simulink library "AEMS_Standard_Library"  (R2016b)
settings: Solver=ode45  StartTime=0.0  StopTime=10.0  RelTol=1e-3
undefined symbols (not defined in the file or in its folder): BkPY, carto, Cbx_extegr, Cbx_lpegrsys, Cbx_portegr, Cnx_bnk_nr_conf, Cnx_cyl_nr_conf, ConfigManagement, configuration_management, Cxx_dcm_io_tmr_end_xxxx, Cxx_dcm_rt_tmr_end, Cxx_DID_xxxx_IO_max, Cxx_DID_xxxx_IO_min, Cxx_egrhsofs, Cxx_vmaniegi, DEM_DEBOUNCE_FREEZE, DEM_DTR_CTL_INVISIBLE, DEM_DTR_CTL_NORMAL, Dem_DtrId2_XXX, Dem_DtrId3_XXX, Dem_DtrId4_XXX, Dem_DtrId5_XXX, Dem_DtrId6_XXX, Dem_DtrId7_XXX, Dem_DtrId8_XXX, Dem_DtrId9_XXX, Dem_DtrId_XXX, Dem_EnableConditionId2_XXX, Dem_EnableConditionId3_XXX, Dem_EnableConditionId4_XXX, Dem_EnableConditionId5_XXX, Dem_EnableConditionId6_XXX, Dem_EnableConditionId7_XXX, Dem_EnableConditionId8_XXX, Dem_EnableConditionId_XXX, Dem_EventId, Dem_EventId2_XXX, Dem_EventId3_XXX, Dem_EventId4_XXX, Dem_EventId5_XXX, Dem_EventId6_XXX, Dem_EventId7_XXX, Dem_EventId8_XXX, Dem_EventId9_XXX, Dem_EventId_Device_Faulttype, Dem_EventId_XXX, DEM_IUMPR_GENERAL_DENOMINATOR, DEM_OPCYC_IGNITION, Dem_RatioId2_XXX, Dem_RatioId3_XXX, Dem_RatioId4_XXX, Dem_RatioId5_XXX, Dem_RatioId6_XXX, Dem_RatioId7_XXX, Dem_RatioId8_XXX, Dem_RatioId_XXX, Dem_StorageConditionId2_XXX, Dem_StorageConditionId3_XXX, Dem_StorageConditionId4_XXX, Dem_StorageConditionId5_XXX ... (+65)
libraries: AEMS_Standard_Library x477, simulink x2
(part 23 of 39)

== system AEMS_Standard_Library/SUB/AEMS_DEM_REP_IUMPR_8D ==
  denlock_status : Inport
  faultdetect_trigger : Inport  Port=2
  AEMS_EDGE_FALLING : AEMS_Standard_Library/EDGE/AEMS_EDGE_FALLING  Tag=[LIB]  init=false
      settings: AttributesFormatString=|
      | %<MaskType>
      | Initial Value : %<init>
  AEMS_EDGE_RISING1 : AEMS_Standard_Library/EDGE/AEMS_EDGE_RISING  Tag=[LIB]  init=false
      settings: AttributesFormatString=|
      | %<MaskType>
      | Initial Value : %<init>
  AEMS_EDGE_RISING2 : AEMS_Standard_Library/EDGE/AEMS_EDGE_RISING  Tag=[LIB]  init=false
      settings: AttributesFormatString=|
      | %<MaskType>
      | Initial Value : %<init>
  Dem_RepIUMPRDenLock_Call1 : Subsystem  TreatAsAtomicUnit=on
  Dem_RepIUMPRDenLock_Call2 : Subsystem  TreatAsAtomicUnit=on
  Dem_RepIUMPRDenLock_Call3 : Subsystem  TreatAsAtomicUnit=on
  Dem_RepIUMPRDenLock_Call4 : Subsystem  TreatAsAtomicUnit=on
  Dem_RepIUMPRDenLock_Call5 : Subsystem  TreatAsAtomicUnit=on
  Dem_RepIUMPRDenLock_Call6 : Subsystem  TreatAsAtomicUnit=on
  Dem_RepIUMPRDenLock_Call7 : Subsystem  TreatAsAtomicUnit=on
  Dem_RepIUMPRDenLock_Call8 : Subsystem  TreatAsAtomicUnit=on
  Dem_RepIUMPRDenRelease_Call1 : Subsystem  TreatAsAtomicUnit=on
  Dem_RepIUMPRDenRelease_Call2 : Subsystem  TreatAsAtomicUnit=on
  Dem_RepIUMPRDenRelease_Call3 : Subsystem  TreatAsAtomicUnit=on
  Dem_RepIUMPRDenRelease_Call4 : Subsystem  TreatAsAtomicUnit=on
  Dem_RepIUMPRDenRelease_Call5 : Subsystem  TreatAsAtomicUnit=on
  Dem_RepIUMPRDenRelease_Call6 : Subsystem  TreatAsAtomicUnit=on
  Dem_RepIUMPRDenRelease_Call7 : Subsystem  TreatAsAtomicUnit=on
  Dem_RepIUMPRDenRelease_Call8 : Subsystem  TreatAsAtomicUnit=on
  Dem_RepIUMPRFaultDetect_Call1 : Subsystem  TreatAsAtomicUnit=on
  Dem_RepIUMPRFaultDetect_Call2 : Subsystem  TreatAsAtomicUnit=on
  Dem_RepIUMPRFaultDetect_Call3 : Subsystem  TreatAsAtomicUnit=on
  Dem_RepIUMPRFaultDetect_Call4 : Subsystem  TreatAsAtomicUnit=on
  Dem_RepIUMPRFaultDetect_Call5 : Subsystem  TreatAsAtomicUnit=on
  Dem_RepIUMPRFaultDetect_Call6 : Subsystem  TreatAsAtomicUnit=on
  Dem_RepIUMPRFaultDetect_Call7 : Subsystem  TreatAsAtomicUnit=on
  Dem_RepIUMPRFaultDetect_Call8 : Subsystem  TreatAsAtomicUnit=on
  Demux : Demux  Outputs=8
  Demux1 : Demux  Outputs=8
  Demux2 : Demux  Outputs=8
  wires:
  AEMS_EDGE_RISING1/1 -> Demux1/1  "denlock_call"
  AEMS_EDGE_RISING2/1 -> Demux/1  "faultdetect_call"
  AEMS_EDGE_FALLING/1 -> Demux2/1  "denrelease_call"
  Demux2/8 -> Dem_RepIUMPRDenRelease_Call8/Enable  "denrelease_call8"
  Demux2/7 -> Dem_RepIUMPRDenRelease_Call7/Enable  "denrelease_call7"
  Demux2/6 -> Dem_RepIUMPRDenRelease_Call6/Enable  "denrelease_call6"
  Demux2/5 -> Dem_RepIUMPRDenRelease_Call5/Enable  "denrelease_call5"
  Demux2/4 -> Dem_RepIUMPRDenRelease_Call4/Enable  "denrelease_call4"
  Demux2/3 -> Dem_RepIUMPRDenRelease_Call3/Enable  "denrelease_call3"
  Demux2/2 -> Dem_RepIUMPRDenRelease_Call2/Enable  "denrelease_call2"
  Demux2/1 -> Dem_RepIUMPRDenRelease_Call1/Enable  "denrelease_call1"
  Demux1/8 -> Dem_RepIUMPRDenLock_Call8/Enable  "denlock_call8"
  Demux1/7 -> Dem_RepIUMPRDenLock_Call7/Enable  "denlock_call7"
  Demux1/6 -> Dem_RepIUMPRDenLock_Call6/Enable  "denlock_call6"
  Demux1/5 -> Dem_RepIUMPRDenLock_Call5/Enable  "denlock_call5"
  Demux1/4 -> Dem_RepIUMPRDenLock_Call4/Enable  "denlock_call4"
  Demux1/3 -> Dem_RepIUMPRDenLock_Call3/Enable  "denlock_call3"
  Demux1/2 -> Dem_RepIUMPRDenLock_Call2/Enable  "denlock_call2"
  Demux1/1 -> Dem_RepIUMPRDenLock_Call1/Enable  "denlock_call1"
  denlock_status/1 -> AEMS_EDGE_RISING1/1, AEMS_EDGE_FALLING/1  "denlock_status"
  Demux/8 -> Dem_RepIUMPRFaultDetect_Call8/Enable  "faultdetect_call8"
  Demux/7 -> Dem_RepIUMPRFaultDetect_Call7/Enable  "faultdetect_call7"
  Demux/6 -> Dem_RepIUMPRFaultDetect_Call6/Enable  "faultdetect_call6"
  Demux/5 -> Dem_RepIUMPRFaultDetect_Call5/Enable  "faultdetect_call5"
  Demux/4 -> Dem_RepIUMPRFaultDetect_Call4/Enable  "faultdetect_call4"
  Demux/3 -> Dem_RepIUMPRFaultDetect_Call3/Enable  "faultdetect_call3"
  Demux/2 -> Dem_RepIUMPRFaultDetect_Call2/Enable  "faultdetect_call2"
  Demux/1 -> Dem_RepIUMPRFaultDetect_Call1/Enable  "faultdetect_call1"
  faultdetect_trigger/1 -> AEMS_EDGE_RISING2/1  "faultdetect_trigger"

== system AEMS_Standard_Library/SUB/AEMS_DEM_REP_IUMPR_DEN_RELEASE_1D ==
  denlock_status : Inport  OutDataTypeStr=boolean  PortDimensions=1
  AEMS_EDGE_RISING1 : AEMS_Standard_Library/EDGE/AEMS_EDGE_RISING  Tag=[LIB]  init=false
      settings: AttributesFormatString=|
      | %<MaskType>
      | Initial Value : %<init>
  Dem_RepIUMPRDenRelease_call : Subsystem  TreatAsAtomicUnit=on
  wires:
  denlock_status/1 -> AEMS_EDGE_RISING1/1  "denlock_status"
  AEMS_EDGE_RISING1/1 -> Dem_RepIUMPRDenRelease_call/Enable  "denrelease_call"

== system AEMS_Standard_Library/SUB/AEMS_DEM_REP_IUMPR_DEN_RELEASE_2D ==
  denlock_status : Inport  OutDataTypeStr=boolean
  AEMS_EDGE_RISING2 : AEMS_Standard_Library/EDGE/AEMS_EDGE_RISING  Tag=[LIB]  init=false
      settings: AttributesFormatString=|
      | %<MaskType>
      | Initial Value : %<init>
  Dem_RepIUMPRDenRelease_call1 : Subsystem  TreatAsAtomicUnit=on
  Dem_RepIUMPRDenRelease_call2 : Subsystem  TreatAsAtomicUnit=on
  Demux1 : Demux  Outputs=2
  wires:
  Demux1/2 -> Dem_RepIUMPRDenRelease_call2/Enable  "denrelease_call2"
  Demux1/1 -> Dem_RepIUMPRDenRelease_call1/Enable  "denrelease_call1"
  AEMS_EDGE_RISING2/1 -> Demux1/1  "denrelease_call"
  denlock_status/1 -> AEMS_EDGE_RISING2/1  "denlock_status"

== system AEMS_Standard_Library/SUB/AEMS_DEM_REP_IUMPR_DEN_RELEASE_8D ==
  denlock_status : Inport  OutDataTypeStr=boolean
  AEMS_EDGE_RISING1 : AEMS_Standard_Library/EDGE/AEMS_EDGE_RISING  Tag=[LIB]  init=false
      settings: AttributesFormatString=|
      | %<MaskType>
      | Initial Value : %<init>
  Dem_RepIUMPRDenRelease_call1 : Subsystem  TreatAsAtomicUnit=on
  Dem_RepIUMPRDenRelease_call2 : Subsystem  TreatAsAtomicUnit=on
  Dem_RepIUMPRDenRelease_call3 : Subsystem  TreatAsAtomicUnit=on
  Dem_RepIUMPRDenRelease_call4 : Subsystem  TreatAsAtomicUnit=on
  Dem_RepIUMPRDenRelease_call5 : Subsystem  TreatAsAtomicUnit=on
  Dem_RepIUMPRDenRelease_call6 : Subsystem  TreatAsAtomicUnit=on
  Dem_RepIUMPRDenRelease_call7 : Subsystem  TreatAsAtomicUnit=on
  Dem_RepIUMPRDenRelease_call8 : Subsystem  TreatAsAtomicUnit=on
  Demux1 : Demux  Outputs=8
  wires:
  AEMS_EDGE_RISING1/1 -> Demux1/1  "denrelease_call"
  Demux1/8 -> Dem_RepIUMPRDenRelease_call8/Enable  "denrelease_call8"
  Demux1/7 -> Dem_RepIUMPRDenRelease_call7/Enable  "denrelease_call7"
  Demux1/6 -> Dem_RepIUMPRDenRelease_call6/Enable  "denrelease_call6"
  Demux1/5 -> Dem_RepIUMPRDenRelease_call5/Enable  "denrelease_call5"
  Demux1/4 -> Dem_RepIUMPRDenRelease_call4/Enable  "denrelease_call4"
  Demux1/3 -> Dem_RepIUMPRDenRelease_call3/Enable  "denrelease_call3"
  Demux1/2 -> Dem_RepIUMPRDenRelease_call2/Enable  "denrelease_call2"
  Demux1/1 -> Dem_RepIUMPRDenRelease_call1/Enable  "denrelease_call1"
  denlock_status/1 -> AEMS_EDGE_RISING1/1  "denlock_status"

== system AEMS_Standard_Library/SUB/AEMS_DEM_REP_IUMPR_FAULTDETECT_1D ==
  faultdetect_trigger : Inport  OutDataTypeStr=boolean  PortDimensions=1
  AEMS_EDGE_RISING : AEMS_Standard_Library/EDGE/AEMS_EDGE_RISING  Tag=[LIB]  init=false
      settings: AttributesFormatString=|
      | %<MaskType>
      | Initial Value : %<init>
  Dem_RepIUMPRFaultDetect_call1 : Subsystem  TreatAsAtomicUnit=on
  wires:
  AEMS_EDGE_RISING/1 -> Dem_RepIUMPRFaultDetect_call1/Enable  "faultdetect_call1"
  faultdetect_trigger/1 -> AEMS_EDGE_RISING/1  "faultdetect_trigger"

== system AEMS_Standard_Library/SUB/AEMS_DEM_REP_IUMPR_FAULTDETECT_2D ==
  faultdetect_trigger : Inport  OutDataTypeStr=boolean
  AEMS_EDGE_RISING1 : AEMS_Standard_Library/EDGE/AEMS_EDGE_RISING  Tag=[LIB]  init=false
      settings: AttributesFormatString=|
      | %<MaskType>
      | Initial Value : %<init>
  Dem_RepIUMPRFaultDetect_Call1 : Subsystem  TreatAsAtomicUnit=on
  Dem_RepIUMPRFaultDetect_Call2 : Subsystem  TreatAsAtomicUnit=on
  Demux : Demux  Outputs=2
  wires:
  faultdetect_trigger/1 -> AEMS_EDGE_RISING1/1  "faultdetect_trigger"
  AEMS_EDGE_RISING1/1 -> Demux/1  "faultdetect_call"
  Demux/1 -> Dem_RepIUMPRFaultDetect_Call1/Enable  "faultdetect_call1"
  Demux/2 -> Dem_RepIUMPRFaultDetect_Call2/Enable  "faultdetect_call2"

== system AEMS_Standard_Library/SUB/AEMS_DEM_REP_IUMPR_FAULTDETECT_8D ==
  faultdetect_trigger : Inport  OutDataTypeStr=boolean
  AEMS_EDGE_RISING2 : AEMS_Standard_Library/EDGE/AEMS_EDGE_RISING  Tag=[LIB]  init=false
      settings: AttributesFormatString=|
      | %<MaskType>
      | Initial Value : %<init>
  Dem_RepIUMPRFaultDetect_Call1 : Subsystem  TreatAsAtomicUnit=on
  Dem_RepIUMPRFaultDetect_Call2 : Subsystem  TreatAsAtomicUnit=on
  Dem_RepIUMPRFaultDetect_Call3 : Subsystem  TreatAsAtomicUnit=on
  Dem_RepIUMPRFaultDetect_Call4 : Subsystem  TreatAsAtomicUnit=on
  Dem_RepIUMPRFaultDetect_Call5 : Subsystem  TreatAsAtomicUnit=on
  Dem_RepIUMPRFaultDetect_Call6 : Subsystem  TreatAsAtomicUnit=on
  Dem_RepIUMPRFaultDetect_Call7 : Subsystem  TreatAsAtomicUnit=on
  Dem_RepIUMPRFaultDetect_Call8 : Subsystem  TreatAsAtomicUnit=on
  Demux : Demux  Outputs=8
  wires:
  faultdetect_trigger/1 -> AEMS_EDGE_RISING2/1  "faultdetect_trigger"
  Demux/1 -> Dem_RepIUMPRFaultDetect_Call1/Enable  "faultdetect_call1"
  Demux/2 -> Dem_RepIUMPRFaultDetect_Call2/Enable  "faultdetect_call2"
  Demux/3 -> Dem_RepIUMPRFaultDetect_Call3/Enable  "faultdetect_call3"
  Demux/4 -> Dem_RepIUMPRFaultDetect_Call4/Enable  "faultdetect_call4"
  Demux/5 -> Dem_RepIUMPRFaultDetect_Call5/Enable  "faultdetect_call5"
  Demux/6 -> Dem_RepIUMPRFaultDetect_Call6/Enable  "faultdetect_call6"
  Demux/7 -> Dem_RepIUMPRFaultDetect_Call7/Enable  "faultdetect_call7"
  Demux/8 -> Dem_RepIUMPRFaultDetect_Call8/Enable  "faultdetect_call8"
  AEMS_EDGE_RISING2/1 -> Demux/1  "faultdetect_call"

== system AEMS_Standard_Library/SUB/AEMS_DEM_SETDTR ==
  dtrid : Inport
  test_result : Inport  Port=2
  lower_limit : Inport  Port=3
  upper_limit : Inport  Port=4
  ctrl_val : Inport  Port=5
  Data Type Conversion1 : DataTypeConversion  OutDataTypeStr=uint8
  Ground1 : Ground
  Terminator{,1..5} (6 alike) : Terminator
  wires:
  ctrl_val/1 -> Terminator4/1  "ctrl_val"
  upper_limit/1 -> Terminator3/1  "upper_limit"
  lower_limit/1 -> Terminator2/1  "lower_limit"
  test_result/1 -> Terminator1/1  "test_result"
  dtrid/1 -> Terminator/1  "dtrid"
  Ground1/1 -> Data Type Conversion1/1
  Data Type Conversion1/1 -> Terminator5/1  "Std_ReturnType"

== system AEMS_Standard_Library/SUB/AEMS_DEM_SETENABLECONDITION ==
  EnableConditionID : Inport
  ConditionFulfilled : Inport  Port=2
  Data Type Conversion1 : DataTypeConversion  OutDataTypeStr=uint8
  Ground1 : Ground
  Terminator : Terminator
  Terminator1 : Terminator
  Terminator2 : Terminator
  wires:
  EnableConditionID/1 -> Terminator/1  "enableconditionid"
  ConditionFulfilled/1 -> Terminator1/1  "conditionfulfilled"
  Ground1/1 -> Data Type Conversion1/1
  Data Type Conversion1/1 -> Terminator2/1  "Std_ReturnType"

== system AEMS_Standard_Library/SUB/AEMS_DEM_SETEVENTAVAILABLE ==
  eventid : Inport
  availablestatus : Inport  Port=2
  Data Type Conversion1 : DataTypeConversion  OutDataTypeStr=uint8
  Ground1 : Ground
  Terminator : Terminator
  Terminator1 : Terminator
  Terminator2 : Terminator
  wires:
  Data Type Conversion1/1 -> Terminator2/1  "Std_ReturnType"
  Ground1/1 -> Data Type Conversion1/1
  availablestatus/1 -> Terminator1/1  "availablestatus"
  eventid/1 -> Terminator/1  "eventid"

== system AEMS_Standard_Library/SUB/AEMS_DEM_SETEVENTDISABLED ==
  eventid : Inport
  Data Type Conversion1 : DataTypeConversion  OutDataTypeStr=uint8
  Ground1 : Ground
  Terminator : Terminator
  Terminator1 : Terminator
  wires:
  eventid/1 -> Terminator/1  "eventid"
  Ground1/1 -> Data Type Conversion1/1
  Data Type Conversion1/1 -> Terminator1/1  "Std_ReturnType"

== system AEMS_Standard_Library/SUB/AEMS_DEM_SETEVENTSTATUS ==
  eventid : Inport
      settings: AttributesFormatString=<tsample=%<SampleTime>>
  eventstatus : Inport  Port=2
      settings: AttributesFormatString=<tsample=%<SampleTime>>
  Data Type Conversion1 : DataTypeConversion  OutDataTypeStr=uint8
  Ground1 : Ground
  Terminator : Terminator
  Terminator1 : Terminator
  Terminator2 : Terminator
  wires:
  eventstatus/1 -> Terminator1/1  "eventstatus"
  eventid/1 -> Terminator/1  "eventid"
  Ground1/1 -> Data Type Conversion1/1
  Data Type Conversion1/1 -> Terminator2/1  "Std_ReturnType"

== system AEMS_Standard_Library/SUB/AEMS_DEM_SETIUMPRDENCONDITION ==
  condition_id : Inport
  condition_status : Inport  Port=2
  Data Type Conversion1 : DataTypeConversion  OutDataTypeStr=uint8
  Ground1 : Ground
  Terminator : Terminator
  Terminator1 : Terminator
  Terminator2 : Terminator
  wires:
  condition_status/1 -> Terminator1/1  "condition_status"
  condition_id/1 -> Terminator/1  "condition_id"
  Ground1/1 -> Data Type Conversion1/1
  Data Type Conversion1/1 -> Terminator2/1  "Std_ReturnType"

== system AEMS_Standard_Library/SUB/AEMS_DEM_SETOPERATIONCYCLESTATE ==
  operation_cycleid : Inport
  cycle_state : Inport  Port=2
  Data Type Conversion1 : DataTypeConversion  OutDataTypeStr=uint8
  Ground1 : Ground
  Terminator : Terminator
  Terminator1 : Terminator
  Terminator2 : Terminator
  wires:
  cycle_state/1 -> Terminator1/1  "cycle_state"
  operation_cycleid/1 -> Terminator/1  "operation_cycleid"
  Ground1/1 -> Data Type Conversion1/1
  Data Type Conversion1/1 -> Terminator2/1  "Std_ReturnType"

== system AEMS_Standard_Library/SUB/AEMS_DEM_SETPFCCYCLEQUALIFIED ==
  Data Type Conversion1 : DataTypeConversion  OutDataTypeStr=uint8
  Ground1 : Ground
  Terminator1 : Terminator
  wires:
  Ground1/1 -> Data Type Conversion1/1
  Data Type Conversion1/1 -> Terminator1/1  "Std_ReturnType"

== system AEMS_Standard_Library/SUB/AEMS_DEM_SETSTORAGECONDITION ==
  StorageConditionID : Inport
  ConditionFulfilled : Inport  Port=2
  Data Type Conversion1 : DataTypeConversion  OutDataTypeStr=uint8
  Ground1 : Ground
  Terminator : Terminator
  Terminator1 : Terminator
  Terminator2 : Terminator
  wires:
  ConditionFulfilled/1 -> Terminator1/1  "ConditionFulfilled"
  StorageConditionID/1 -> Terminator/1  "StorageConditionID"
  Ground1/1 -> Data Type Conversion1/1
  Data Type Conversion1/1 -> Terminator2/1  "Std_ReturnType"

== system AEMS_Standard_Library/SUB/AEMS_DEM_SET_DTR_1DS ==
  set_flag : Inport  Interpolate=off
  testresult : Inport  Port=2  Interpolate=off
  lowerlimit : Inport  Port=3  Interpolate=off
  upperlimit : Inport  Port=4  Interpolate=off
  ctrl_flag : Inport  Port=5  Interpolate=off
  Dem_SetDTR_Call : Subsystem
  deadzone : Subsystem
  wires:
  ctrl_flag/1 -> Dem_SetDTR_Call/4(ctrl_flag)  "ctrl_flag"
  set_flag/1 -> Dem_SetDTR_Call/Enable  "set_flag"
  testresult/1 -> deadzone/1(testresult)  "testresult"
  lowerlimit/1 -> Dem_SetDTR_Call/2(lowerlimit), deadzone/2(lowerlimit)  "lowerlimit"
  upperlimit/1 -> deadzone/3(upperlimit), Dem_SetDTR_Call/3(upperlimit)  "upperlimit"
  deadzone/1(customresult) -> Dem_SetDTR_Call/1(customresult)

== system AEMS_Standard_Library/SUB/AEMS_DEM_SET_DTR_1DU ==
  set_flag : Inport  OutDataTypeStr=boolean  PortDimensions=1  Interpolate=off
  testresult : Inport  Port=2  OutDataTypeStr=uint16  PortDimensions=1  Interpolate=off
  lowerlimit : Inport  Port=3  OutDataTypeStr=uint16  PortDimensions=1  Interpolate=off
  upperlimit : Inport  Port=4  OutDataTypeStr=uint16  PortDimensions=1  Interpolate=off
  ctrl_flag : Inport  Port=5  OutDataTypeStr=boolean  PortDimensions=1  Interpolate=off
  Dem_SetDTR_Call : Subsystem
  wires:
  upperlimit/1 -> Dem_SetDTR_Call/3(upperlimit)  "upperlimit"
  lowerlimit/1 -> Dem_SetDTR_Call/2(lowerlimit)  "lowerlimit"
  testresult/1 -> Dem_SetDTR_Call/1(testresult)  "testresult"
  set_flag/1 -> Dem_SetDTR_Call/Enable  "set_flag"
  ctrl_flag/1 -> Dem_SetDTR_Call/4(ctrl_flag)  "ctrl_flag"

== system AEMS_Standard_Library/SUB/AEMS_DEM_SET_DTR_2DS ==
  set_flag : Inport  Interpolate=off
  testresult : Inport  Port=2  Interpolate=off
  lowerlimit : Inport  Port=3  Interpolate=off
  upperlimit : Inport  Port=4  Interpolate=off
  ctrl_flag : Inport  Port=5  Interpolate=off
  Deadzone : Subsystem
  Dem_SetDTR_Call1 : Subsystem
  Dem_SetDTR_Call2 : Subsystem
  Demux{1,3..6} (5 alike) : Demux  Outputs=2
  wires:
  Demux6/2 -> Dem_SetDTR_Call2/3(upperlimit2)  "upperlimit2"
  Demux5/2 -> Dem_SetDTR_Call2/2(lowerlimit2)  "lowerlimit2"
  Demux4/2 -> Dem_SetDTR_Call2/1(customresult2)  "customresult2"
  Demux6/1 -> Dem_SetDTR_Call1/3(upperlimit1)  "upperlimit1"
  Demux5/1 -> Dem_SetDTR_Call1/2(lowerlimit1)  "lowerlimit1"
  Demux4/1 -> Dem_SetDTR_Call1/1(customresult1)  "customresult1"
  Demux3/2 -> Dem_SetDTR_Call2/Enable  "set_flag2"
  Demux3/1 -> Dem_SetDTR_Call1/Enable  "set_flag1"
  set_flag/1 -> Demux3/1  "set_flag"
  upperlimit/1 -> Deadzone/3(upperlimit), Demux6/1  "upperlimit"
  lowerlimit/1 -> Deadzone/2(lowerlimit), Demux5/1  "lowerlimit"
  Deadzone/1(customresult) -> Demux4/1
  testresult/1 -> Deadzone/1(testresult)  "testresult"
  Demux1/1 -> Dem_SetDTR_Call1/4(ctrl_flag1)  "ctrl_flag1"
  Demux1/2 -> Dem_SetDTR_Call2/4(ctrl_flag2)  "ctrl_flag2"
  ctrl_flag/1 -> Demux1/1  "ctrl_flag"

== system AEMS_Standard_Library/SUB/AEMS_DEM_SET_DTR_2DU ==
  set_flag : Inport  Interpolate=off
  testresult : Inport  Port=2  Interpolate=off
  lowerlimit : Inport  Port=3  Interpolate=off
  upperlimit : Inport  Port=4  Interpolate=off
  ctrl_flag : Inport  Port=5  Interpolate=off
  Dem_SetDTR_Call1 : Subsystem
  Dem_SetDTR_Call2 : Subsystem
  Demux{1,3..6} (5 alike) : Demux  Outputs=2
  wires:
  Demux1/2 -> Dem_SetDTR_Call2/4(ctrl_flag2)  "ctrl_flag2"
  Demux1/1 -> Dem_SetDTR_Call1/4(ctrl_flag1)  "ctrl_flag1"
  ctrl_flag/1 -> Demux1/1  "ctrl_flag"
  set_flag/1 -> Demux3/1  "set_flag"
  testresult/1 -> Demux4/1  "testresult"
  lowerlimit/1 -> Demux5/1  "lowerlimit"
  upperlimit/1 -> Demux6/1  "upperlimit"
  Demux3/1 -> Dem_SetDTR_Call1/Enable  "set_flag1"
  Demux3/2 -> Dem_SetDTR_Call2/Enable  "set_flag2"
  Demux4/1 -> Dem_SetDTR_Call1/1(testresult1)  "testresult1"
  Demux5/1 -> Dem_SetDTR_Call1/2(lowerlimit1)  "lowerlimit1"
  Demux6/1 -> Dem_SetDTR_Call1/3(upperlimit1)  "upperlimit1"
  Demux4/2 -> Dem_SetDTR_Call2/1(testresult2)  "testresult2"
  Demux5/2 -> Dem_SetDTR_Call2/2(lowerlimit2)  "lowerlimit2"
  Demux6/2 -> Dem_SetDTR_Call2/3(upperlimit2)  "upperlimit2"

== system AEMS_Standard_Library/SUB/AEMS_DEM_SET_DTR_8DS ==
  set_flag : Inport  Interpolate=off
  testresult : Inport  Port=2  Interpolate=off
  lowerlimit : Inport  Port=3  Interpolate=off
  upperlimit : Inport  Port=4  Interpolate=off
  ctrl_flag : Inport  Port=5  Interpolate=off
  Deadzone : Subsystem
  Dem_SetDTR_Call1 : Subsystem
  Dem_SetDTR_Call2 : Subsystem
  Dem_SetDTR_Call3 : Subsystem
  Dem_SetDTR_Call4 : Subsystem
  Dem_SetDTR_Call5 : Subsystem
  Dem_SetDTR_Call6 : Subsystem
  Dem_SetDTR_Call7 : Subsystem
  Dem_SetDTR_Call8 : Subsystem
  Demux{1..5} (5 alike) : Demux  Outputs=8
  wires:
  Demux3/5 -> Dem_SetDTR_Call5/Enable  "set_flag5"
  Demux2/8 -> Dem_SetDTR_Call8/3(upperlimit8)  "upperlimit8"
  Demux2/7 -> Dem_SetDTR_Call7/3(upperlimit7)  "upperlimit7"
  Demux2/6 -> Dem_SetDTR_Call6/3(upperlimit6)  "upperlimit6"
  Demux2/5 -> Dem_SetDTR_Call5/3(upperlimit5)  "upperlimit5"
  Demux2/4 -> Dem_SetDTR_Call4/3(upperlimit4)  "upperlimit4"
  Demux2/3 -> Dem_SetDTR_Call3/3(upperlimit3)  "upperlimit3"
  Demux2/2 -> Dem_SetDTR_Call2/3(upperlimit2)  "upperlimit2"
  Demux2/1 -> Dem_SetDTR_Call1/3(upperlimit1)  "upperlimit1"
  Demux1/8 -> Dem_SetDTR_Call8/2(lowerlimit8)  "lowerlimit8"
  Demux1/7 -> Dem_SetDTR_Call7/2(lowerlimit7)  "lowerlimit7"
  Demux1/6 -> Dem_SetDTR_Call6/2(lowerlimit6)  "lowerlimit6"
  Demux1/5 -> Dem_SetDTR_Call5/2(lowerlimit5)  "lowerlimit5"
  Demux1/4 -> Dem_SetDTR_Call4/2(lowerlimit4)  "lowerlimit4"
  Demux1/3 -> Dem_SetDTR_Call3/2(lowerlimit3)  "lowerlimit3"
  Demux1/2 -> Dem_SetDTR_Call2/2(lowerlimit2)  "lowerlimit2"
  Demux1/1 -> Dem_SetDTR_Call1/2(lowerlimit1)  "lowerlimit1"
  Demux4/8 -> Dem_SetDTR_Call8/1(customresult8)  "customresult8"
  Demux4/7 -> Dem_SetDTR_Call7/1(customresult7)  "customresult7"
  Demux4/6 -> Dem_SetDTR_Call6/1(customresult6)  "customresult6"
  Demux4/5 -> Dem_SetDTR_Call5/1(customresult5)  "customresult5"
  Demux4/4 -> Dem_SetDTR_Call4/1(customresult4)  "customresult4"
  Demux4/3 -> Dem_SetDTR_Call3/1(customresult3)  "customresult3"
  Demux4/2 -> Dem_SetDTR_Call2/1(customresult2)  "customresult2"
  Demux4/1 -> Dem_SetDTR_Call1/1(customresult1)  "customresult1"
  Demux3/8 -> Dem_SetDTR_Call8/Enable  "set_flag8"
  Demux3/7 -> Dem_SetDTR_Call7/Enable  "set_flag7"
  Demux3/6 -> Dem_SetDTR_Call6/Enable  "set_flag6"
  Demux3/4 -> Dem_SetDTR_Call4/Enable  "set_flag4"
  Demux3/3 -> Dem_SetDTR_Call3/Enable  "set_flag3"
  Demux3/2 -> Dem_SetDTR_Call2/Enable  "set_flag2"
  Demux3/1 -> Dem_SetDTR_Call1/Enable  "set_flag1"
  Deadzone/1(customresult) -> Demux4/1
  upperlimit/1 -> Deadzone/3(upperlimit), Demux2/1  "upperlimit"
  lowerlimit/1 -> Deadzone/2(lowerlimit), Demux1/1  "lowerlimit"
  testresult/1 -> Deadzone/1(testresult)  "testresult"
  set_flag/1 -> Demux3/1  "set_flag"
  ctrl_flag/1 -> Demux5/1  "ctrl_flag"
  Demux5/1 -> Dem_SetDTR_Call1/4(ctrl_flag1)  "ctrl_flag1"
  Demux5/2 -> Dem_SetDTR_Call2/4(ctrl_flag2)  "ctrl_flag2"
  Demux5/3 -> Dem_SetDTR_Call3/4(ctrl_flag3)  "ctrl_flag3"
  Demux5/4 -> Dem_SetDTR_Call4/4(ctrl_flag4)  "ctrl_flag4"
  Demux5/5 -> Dem_SetDTR_Call5/4(ctrl_flag5)  "ctrl_flag5"
  Demux5/6 -> Dem_SetDTR_Call6/4(ctrl_flag6)  "ctrl_flag6"
  Demux5/7 -> Dem_SetDTR_Call7/4(ctrl_flag7)  "ctrl_flag7"
  Demux5/8 -> Dem_SetDTR_Call8/4(ctrl_flag8)  "ctrl_flag8"

== system AEMS_Standard_Library/SUB/AEMS_DEM_SET_DTR_8DU ==
  set_flag : Inport  Interpolate=off
  testresult : Inport  Port=2  Interpolate=off
  lowerlimit : Inport  Port=3  Interpolate=off
  upperlimit : Inport  Port=4  Interpolate=off
  ctrl_flag : Inport  Port=5  Interpolate=off
  Dem_SetDTR_Call1 : Subsystem
  Dem_SetDTR_Call2 : Subsystem
  Dem_SetDTR_Call3 : Subsystem
  Dem_SetDTR_Call4 : Subsystem
  Dem_SetDTR_Call5 : Subsystem
  Dem_SetDTR_Call6 : Subsystem
  Dem_SetDTR_Call7 : Subsystem
  Dem_SetDTR_Call8 : Subsystem
  Demux{1..5} (5 alike) : Demux  Outputs=8
  wires:
  upperlimit/1 -> Demux2/1  "upperlimit"
  lowerlimit/1 -> Demux1/1  "lowerlimit"
  testresult/1 -> Demux4/1  "testresult"
  set_flag/1 -> Demux3/1  "set_flag"
  ctrl_flag/1 -> Demux5/1  "ctrl_flag"
  Demux3/1 -> Dem_SetDTR_Call1/Enable  "set_flag1"
  Demux3/2 -> Dem_SetDTR_Call2/Enable  "set_flag2"
  Demux3/3 -> Dem_SetDTR_Call3/Enable  "set_flag3"
  Demux3/4 -> Dem_SetDTR_Call4/Enable  "set_flag4"
  Demux3/5 -> Dem_SetDTR_Call5/Enable  "set_flag5"
  Demux3/6 -> Dem_SetDTR_Call6/Enable  "set_flag6"
  Demux3/7 -> Dem_SetDTR_Call7/Enable  "set_flag7"
  Demux3/8 -> Dem_SetDTR_Call8/Enable  "set_flag8"
  Demux4/8 -> Dem_SetDTR_Call8/1(testresult8)  "testresult8"
  Demux4/1 -> Dem_SetDTR_Call1/1(testresult1)  "testresult1"
  Demux4/2 -> Dem_SetDTR_Call2/1(testresult2)  "testresult2"
  Demux4/3 -> Dem_SetDTR_Call3/1(testresult3)  "testresult3"
  Demux4/4 -> Dem_SetDTR_Call4/1(testresult4)  "testresult4"
  Demux4/5 -> Dem_SetDTR_Call5/1(testresult5)  "testresult5"
  Demux4/6 -> Dem_SetDTR_Call6/1(testresult6)  "testresult6"
  Demux4/7 -> Dem_SetDTR_Call7/1(testresult7)  "testresult7"
  Demux1/1 -> Dem_SetDTR_Call1/2(lowerlimit1)  "lowerlimit1"
  Demux1/2 -> Dem_SetDTR_Call2/2(lowerlimit2)  "lowerlimit2"
  Demux1/3 -> Dem_SetDTR_Call3/2(lowerlimit3)  "lowerlimit3"
  Demux1/4 -> Dem_SetDTR_Call4/2(lowerlimit4)  "lowerlimit4"
  Demux1/5 -> Dem_SetDTR_Call5/2(lowerlimit5)  "lowerlimit5"
  Demux1/6 -> Dem_SetDTR_Call6/2(lowerlimit6)  "lowerlimit6"
  Demux1/7 -> Dem_SetDTR_Call7/2(lowerlimit7)  "lowerlimit7"
  Demux1/8 -> Dem_SetDTR_Call8/2(lowerlimit8)  "lowerlimit8"
  Demux2/1 -> Dem_SetDTR_Call1/3(upperlimit1)  "upperlimit1"
  Demux2/2 -> Dem_SetDTR_Call2/3(upperlimit2)  "upperlimit2"
  Demux2/3 -> Dem_SetDTR_Call3/3(upperlimit3)  "upperlimit3"
  Demux2/4 -> Dem_SetDTR_Call4/3(upperlimit4)  "upperlimit4"
  Demux2/5 -> Dem_SetDTR_Call5/3(upperlimit5)  "upperlimit5"
  Demux2/6 -> Dem_SetDTR_Call6/3(upperlimit6)  "upperlimit6"
  Demux2/7 -> Dem_SetDTR_Call7/3(upperlimit7)  "upperlimit7"
  Demux2/8 -> Dem_SetDTR_Call8/3(upperlimit8)  "upperlimit8"
  Demux5/1 -> Dem_SetDTR_Call1/4(ctrl_flag1)  "ctrl_flag1"
  Demux5/2 -> Dem_SetDTR_Call2/4(ctrl_flag2)  "ctrl_flag2"
  Demux5/3 -> Dem_SetDTR_Call3/4(ctrl_flag3)  "ctrl_flag3"
  Demux5/4 -> Dem_SetDTR_Call4/4(ctrl_flag4)  "ctrl_flag4"
  Demux5/5 -> Dem_SetDTR_Call5/4(ctrl_flag5)  "ctrl_flag5"
  Demux5/6 -> Dem_SetDTR_Call6/4(ctrl_flag6)  "ctrl_flag6"
  Demux5/7 -> Dem_SetDTR_Call7/4(ctrl_flag7)  "ctrl_flag7"
  Demux5/8 -> Dem_SetDTR_Call8/4(ctrl_flag8)  "ctrl_flag8"

== system AEMS_Standard_Library/SUB/AEMS_DEM_SET_DTR_9DU ==
  set_flag : Inport  OutDataTypeStr=boolean  PortDimensions=9  Interpolate=off
      settings: AttributesFormatString=<tsample=%<SampleTime>>
  testresult : Inport  Port=2  OutDataTypeStr=uint16  PortDimensions=9  Interpolate=off
      settings: AttributesFormatString=<tsample=%<SampleTime>>
  lowerlimit : Inport  Port=3  OutDataTypeStr=uint16  PortDimensions=9  Interpolate=off
      settings: AttributesFormatString=<tsample=%<SampleTime>>
  upperlimit : Inport  Port=4  OutDataTypeStr=uint16  PortDimensions=9  Interpolate=off
      settings: AttributesFormatString=<tsample=%<SampleTime>>
  ctrl_flag : Inport  Port=5  OutDataTypeStr=boolean  PortDimensions=9  Interpolate=off
      settings: AttributesFormatString=<tsample=%<SampleTime>>
  Dem_SetDTR_Call0 : Subsystem
  Dem_SetDTR_Call1 : Subsystem
  Dem_SetDTR_Call2 : Subsystem
  Dem_SetDTR_Call3 : Subsystem
  Dem_SetDTR_Call4 : Subsystem
  Dem_SetDTR_Call5 : Subsystem
  Dem_SetDTR_Call6 : Subsystem
  Dem_SetDTR_Call7 : Subsystem
  Dem_SetDTR_Call8 : Subsystem
  Demux{1..5} (5 alike) : Demux  Outputs=9
  wires:
  upperlimit/1 -> Demux2/1  "upperlimit"
  lowerlimit/1 -> Demux1/1  "lowerlimit"
  testresult/1 -> Demux4/1  "testresult"
  set_flag/1 -> Demux3/1  "set_flag"
  ctrl_flag/1 -> Demux5/1  "ctrl_flag"
  Demux3/2 -> Dem_SetDTR_Call1/Enable  "set_flag1"
  Demux3/3 -> Dem_SetDTR_Call2/Enable  "set_flag2"
  Demux3/4 -> Dem_SetDTR_Call3/Enable  "set_flag3"
  Demux3/5 -> Dem_SetDTR_Call4/Enable  "set_flag4"
  Demux3/6 -> Dem_SetDTR_Call5/Enable  "set_flag5"
  Demux3/7 -> Dem_SetDTR_Call6/Enable  "set_flag6"
  Demux3/8 -> Dem_SetDTR_Call7/Enable  "set_flag7"
  Demux3/9 -> Dem_SetDTR_Call8/Enable  "set_flag8"
  Demux4/9 -> Dem_SetDTR_Call8/1(testresult8)  "testresult8"
  Demux4/2 -> Dem_SetDTR_Call1/1(testresult1)  "testresult1"
  Demux4/3 -> Dem_SetDTR_Call2/1(testresult2)  "testresult2"
  Demux4/4 -> Dem_SetDTR_Call3/1(testresult3)  "testresult3"
  Demux4/5 -> Dem_SetDTR_Call4/1(testresult4)  "testresult4"
  Demux4/6 -> Dem_SetDTR_Call5/1(testresult5)  "testresult5"
  Demux4/7 -> Dem_SetDTR_Call6/1(testresult6)  "testresult6"
  Demux4/8 -> Dem_SetDTR_Call7/1(testresult7)  "testresult7"
  Demux1/2 -> Dem_SetDTR_Call1/2(lowerlimit1)  "lowerlimit1"
  Demux1/3 -> Dem_SetDTR_Call2/2(lowerlimit2)  "lowerlimit2"
  Demux1/4 -> Dem_SetDTR_Call3/2(lowerlimit3)  "lowerlimit3"
  Demux1/5 -> Dem_SetDTR_Call4/2(lowerlimit4)  "lowerlimit4"
  Demux1/6 -> Dem_SetDTR_Call5/2(lowerlimit5)  "lowerlimit5"
  Demux1/7 -> Dem_SetDTR_Call6/2(lowerlimit6)  "lowerlimit6"
  Demux1/8 -> Dem_SetDTR_Call7/2(lowerlimit7)  "lowerlimit7"
  Demux1/9 -> Dem_SetDTR_Call8/2(lowerlimit8)  "lowerlimit8"
  Demux2/2 -> Dem_SetDTR_Call1/3(upperlimit1)  "upperlimit1"
  Demux2/3 -> Dem_SetDTR_Call2/3(upperlimit2)  "upperlimit2"
  Demux2/4 -> Dem_SetDTR_Call3/3(upperlimit3)  "upperlimit3"
  Demux2/5 -> Dem_SetDTR_Call4/3(upperlimit4)  "upperlimit4"
  Demux2/6 -> Dem_SetDTR_Call5/3(upperlimit5)  "upperlimit5"
  Demux2/7 -> Dem_SetDTR_Call6/3(upperlimit6)  "upperlimit6"
  Demux2/8 -> Dem_SetDTR_Call7/3(upperlimit7)  "upperlimit7"
  Demux2/9 -> Dem_SetDTR_Call8/3(upperlimit8)  "upperlimit8"
  Demux5/2 -> Dem_SetDTR_Call1/4(ctrl_flag1)  "ctrl_flag2"
  Demux5/3 -> Dem_SetDTR_Call2/4(ctrl_flag2)  "ctrl_flag3"
  Demux5/4 -> Dem_SetDTR_Call3/4(ctrl_flag3)  "ctrl_flag4"
  Demux5/5 -> Dem_SetDTR_Call4/4(ctrl_flag4)  "ctrl_flag5"
  Demux5/6 -> Dem_SetDTR_Call5/4(ctrl_flag5)  "ctrl_flag6"
  Demux5/7 -> Dem_SetDTR_Call6/4(ctrl_flag6)  "ctrl_flag7"
  Demux5/8 -> Dem_SetDTR_Call7/4(ctrl_flag7)  "ctrl_flag8"
  Demux5/9 -> Dem_SetDTR_Call8/4(ctrl_flag8)  "ctrl_flag8"
  Demux3/1 -> Dem_SetDTR_Call0/Enable  "set_flag0"
  Demux4/1 -> Dem_SetDTR_Call0/1(testresult0)  "testresult0"
  Demux1/1 -> Dem_SetDTR_Call0/2(lowerlimit0)  "lowerlimit0"
  Demux2/1 -> Dem_SetDTR_Call0/3(upperlimit0)  "upperlimit0"
  Demux5/1 -> Dem_SetDTR_Call0/4(ctrl_flag0)  "ctrl_flag0"

== system AEMS_Standard_Library/SUB/AEMS_DEM_SET_ENBL_COND_1D ==
  conditionfulfilled : Inport
  AEMS_DEM_SETENABLECONDITION : AEMS_Standard_Library/SUB/AEMS_DEM_SETENABLECONDITION  Tag=[LIB]
      settings: AttributesFormatString=%<MaskType>
  EnableConditionId_block : Constant  Value=Dem_EnableConditionId_XXX  OutDataTypeStr=uint8
  wires:
  EnableConditionId_block/1 -> AEMS_DEM_SETENABLECONDITION/1  "enableconditionid"
  conditionfulfilled/1 -> AEMS_DEM_SETENABLECONDITION/2  "conditionfulfilled"

== system AEMS_Standard_Library/SUB/AEMS_DEM_SET_ENBL_COND_2D ==
  conditionfulfilled : Inport
  AEMS_DEM_SETENABLECONDITION1 : AEMS_Standard_Library/SUB/AEMS_DEM_SETENABLECONDITION  Tag=[LIB]
      settings: AttributesFormatString=%<MaskType>
  AEMS_DEM_SETENABLECONDITION2 : AEMS_Standard_Library/SUB/AEMS_DEM_SETENABLECONDITION  Tag=[LIB]
      settings: AttributesFormatString=%<MaskType>
  Demux1 : Demux  Outputs=2
  EnableConditionId_block1 : Constant  Value=Dem_EnableConditionId_XXX  OutDataTypeStr=uint8
  EnableConditionId_block2 : Constant  Value=Dem_EnableConditionId2_XXX  OutDataTypeStr=uint8
  wires:
  conditionfulfilled/1 -> Demux1/1  "conditionfulfilled"
  Demux1/1 -> AEMS_DEM_SETENABLECONDITION1/2  "conditionfulfilled1"
  EnableConditionId_block1/1 -> AEMS_DEM_SETENABLECONDITION1/1  "enableconditionid1"
  EnableConditionId_block2/1 -> AEMS_DEM_SETENABLECONDITION2/1  "enableconditionid2"
  Demux1/2 -> AEMS_DEM_SETENABLECONDITION2/2  "conditionfulfilled2"

== system AEMS_Standard_Library/SUB/AEMS_DEM_SET_ENBL_COND_8D ==
  conditionfulfilled : Inport
  AEMS_DEM_SETENABLECONDITION{1..8} (8 alike) : AEMS_Standard_Library/SUB/AEMS_DEM_SETENABLECONDITION  Tag=[LIB]
      settings: AttributesFormatString=%<MaskType>
  Demux2 : Demux  Outputs=8
  EnableConditionId_block1 : Constant  Value=Dem_EnableConditionId_XXX  OutDataTypeStr=uint8
  EnableConditionId_block2 : Constant  Value=Dem_EnableConditionId2_XXX  OutDataTypeStr=uint8
  EnableConditionId_block3 : Constant  Value=Dem_EnableConditionId3_XXX  OutDataTypeStr=uint8
  EnableConditionId_block4 : Constant  Value=Dem_EnableConditionId4_XXX  OutDataTypeStr=uint8
  EnableConditionId_block5 : Constant  Value=Dem_EnableConditionId5_XXX  OutDataTypeStr=uint8
  EnableConditionId_block6 : Constant  Value=Dem_EnableConditionId6_XXX  OutDataTypeStr=uint8
  EnableConditionId_block7 : Constant  Value=Dem_EnableConditionId7_XXX  OutDataTypeStr=uint8
  EnableConditionId_block8 : Constant  Value=Dem_EnableConditionId8_XXX  OutDataTypeStr=uint8
  wires:
  conditionfulfilled/1 -> Demux2/1  "conditionfulfilled"
  EnableConditionId_block1/1 -> AEMS_DEM_SETENABLECONDITION1/1  "enableconditionid1"
  EnableConditionId_block2/1 -> AEMS_DEM_SETENABLECONDITION2/1  "enableconditionid2"
  EnableConditionId_block4/1 -> AEMS_DEM_SETENABLECONDITION4/1  "enableconditionid4"
  EnableConditionId_block5/1 -> AEMS_DEM_SETENABLECONDITION5/1  "enableconditionid5"
  EnableConditionId_block3/1 -> AEMS_DEM_SETENABLECONDITION3/1  "enableconditionid3"
  EnableConditionId_block6/1 -> AEMS_DEM_SETENABLECONDITION6/1  "enableconditionid6"
  EnableConditionId_block7/1 -> AEMS_DEM_SETENABLECONDITION7/1  "enableconditionid7"
  EnableConditionId_block8/1 -> AEMS_DEM_SETENABLECONDITION8/1  "enableconditionid8"
  Demux2/1 -> AEMS_DEM_SETENABLECONDITION1/2  "conditionfulfilled1"
  Demux2/2 -> AEMS_DEM_SETENABLECONDITION2/2  "conditionfulfilled2"
  Demux2/3 -> AEMS_DEM_SETENABLECONDITION3/2  "conditionfulfilled3"
  Demux2/4 -> AEMS_DEM_SETENABLECONDITION4/2  "conditionfulfilled4"
  Demux2/5 -> AEMS_DEM_SETENABLECONDITION5/2  "conditionfulfilled5"
  Demux2/6 -> AEMS_DEM_SETENABLECONDITION6/2  "conditionfulfilled6"
  Demux2/7 -> AEMS_DEM_SETENABLECONDITION7/2  "conditionfulfilled7"
  Demux2/8 -> AEMS_DEM_SETENABLECONDITION8/2  "conditionfulfilled8"

== system AEMS_Standard_Library/SUB/AEMS_DEM_SET_EVENT_AVL_1D ==
  Constant : Constant  Value=true
  DEM_SET_EVENT_AVL_E : Subsystem  TreatAsAtomicUnit=on
  DEM_SET_EVENT_AVL_UD : UnitDelay  InitialCondition=false  SampleTime=-1
      settings: AttributesFormatString=<initial=%<InitialCondition>>
  Logical Operator : Logic  Operator=NOT  OutDataTypeStr=boolean
  dgnsw : Outport
  wires:
  Logical Operator/1 -> DEM_SET_EVENT_AVL_E/Enable  "trigger_job_1st"
  DEM_SET_EVENT_AVL_UD/1 -> Logical Operator/1
  DEM_SET_EVENT_AVL_E/1(dgnsw) -> dgnsw/1
  Constant/1 -> DEM_SET_EVENT_AVL_UD/1

== system AEMS_Standard_Library/SUB/AEMS_DEM_SET_EVENT_AVL_2D ==
  Constant : Constant  OutDataTypeStr=boolean
  DEM_SET_EVENT_AVL_E : Subsystem  TreatAsAtomicUnit=on
  DEM_SET_EVENT_AVL_UD : UnitDelay  SampleTime=-1
      settings: AttributesFormatString=<initial=%<InitialCondition>>
  Logical Operator : Logic  Operator=NOT  OutDataTypeStr=boolean
  dgnsw : Outport
  wires:
  Constant/1 -> DEM_SET_EVENT_AVL_UD/1
  DEM_SET_EVENT_AVL_UD/1 -> Logical Operator/1
  DEM_SET_EVENT_AVL_E/1(dgnsw) -> dgnsw/1
  Logical Operator/1 -> DEM_SET_EVENT_AVL_E/Enable  "trigger_job_1st"

== system AEMS_Standard_Library/SUB/AEMS_DEM_SET_EVENT_AVL_8D ==
  Constant : Constant  OutDataTypeStr=boolean
  DEM_SET_EVENT_AVL_E : Subsystem  TreatAsAtomicUnit=on
  DEM_SET_EVENT_AVL_UD : UnitDelay  SampleTime=-1
      settings: AttributesFormatString=<initial=%<InitialCondition>>
  Logical Operator : Logic  Operator=NOT  OutDataTypeStr=boolean
  dgnsw : Outport
  wires:
  Logical Operator/1 -> DEM_SET_EVENT_AVL_E/Enable  "trigger_job_1st"
  DEM_SET_EVENT_AVL_E/1(dgnsw) -> dgnsw/1
  DEM_SET_EVENT_AVL_UD/1 -> Logical Operator/1
  Constant/1 -> DEM_SET_EVENT_AVL_UD/1

== system AEMS_Standard_Library/SUB/AEMS_DEM_SET_EVENT_AVL_9D ==
  Constant : Constant  OutDataTypeStr=boolean
  DEM_SET_EVENT_AVL_E : Subsystem
  DEM_SET_EVENT_AVL_UD : UnitDelay  SampleTime=-1
      settings: AttributesFormatString=<initial=%<X0>>
  Logical Operator : Logic  Operator=NOT  OutDataTypeStr=boolean
  dgnsw : Outport
  wires:
  Constant/1 -> DEM_SET_EVENT_AVL_UD/1
  DEM_SET_EVENT_AVL_UD/1 -> Logical Operator/1
  DEM_SET_EVENT_AVL_E/1(dgnsw) -> dgnsw/1
  Logical Operator/1 -> DEM_SET_EVENT_AVL_E/Enable  "trigger_job_1st"

== system AEMS_Standard_Library/SUB/AEMS_DEM_SET_EVENT_DSBL_1D ==
  set_flag : Inport
  Dem_SetEventDisabled_Call : Subsystem  TreatAsAtomicUnit=on
  wires:
  set_flag/1 -> Dem_SetEventDisabled_Call/Enable  "set_flag"

== system AEMS_Standard_Library/SUB/AEMS_DEM_SET_EVENT_DSBL_2D ==
  set_flag : Inport
  Dem_SetEventDisabled_Call1 : Subsystem  TreatAsAtomicUnit=on
  Dem_SetEventDisabled_Call2 : Subsystem  TreatAsAtomicUnit=on
  Demux : Demux  Outputs=2
  wires:
  Demux/2 -> Dem_SetEventDisabled_Call2/Enable  "set_flag2"
  Demux/1 -> Dem_SetEventDisabled_Call1/Enable  "set_flag1"
  set_flag/1 -> Demux/1  "set_flag"

== system AEMS_Standard_Library/SUB/AEMS_DEM_SET_EVENT_DSBL_8D ==
  set_flag : Inport
  Dem_SetEventDisabled_Call1 : Subsystem  TreatAsAtomicUnit=on
  Dem_SetEventDisabled_Call2 : Subsystem  TreatAsAtomicUnit=on
  Dem_SetEventDisabled_Call3 : Subsystem  TreatAsAtomicUnit=on
  Dem_SetEventDisabled_Call4 : Subsystem  TreatAsAtomicUnit=on
  Dem_SetEventDisabled_Call5 : Subsystem  TreatAsAtomicUnit=on
  Dem_SetEventDisabled_Call6 : Subsystem  TreatAsAtomicUnit=on
  Dem_SetEventDisabled_Call7 : Subsystem  TreatAsAtomicUnit=on
  Dem_SetEventDisabled_Call8 : Subsystem  TreatAsAtomicUnit=on
  Demux : Demux  Outputs=8
  wires:
  Demux/8 -> Dem_SetEventDisabled_Call8/Enable  "set_flag8"
  Demux/7 -> Dem_SetEventDisabled_Call7/Enable  "set_flag7"
  Demux/6 -> Dem_SetEventDisabled_Call6/Enable  "set_flag6"
  Demux/5 -> Dem_SetEventDisabled_Call5/Enable  "set_flag5"
  Demux/4 -> Dem_SetEventDisabled_Call4/Enable  "set_flag4"
  Demux/3 -> Dem_SetEventDisabled_Call3/Enable  "set_flag3"
  Demux/2 -> Dem_SetEventDisabled_Call2/Enable  "set_flag2"
  Demux/1 -> Dem_SetEventDisabled_Call1/Enable  "set_flag1"
  set_flag/1 -> Demux/1  "set_flag"

== system AEMS_Standard_Library/SUB/AEMS_DEM_SET_EVENT_DSBL_9D ==
  set_flag : Inport  OutDataTypeStr=boolean  PortDimensions=9
      settings: AttributesFormatString=<tsample=%<SampleTime>>
  Dem_SetEventDisabled_Call0 : Subsystem  TreatAsAtomicUnit=on
  Dem_SetEventDisabled_Call1 : Subsystem  TreatAsAtomicUnit=on
  Dem_SetEventDisabled_Call2 : Subsystem  TreatAsAtomicUnit=on
  Dem_SetEventDisabled_Call3 : Subsystem  TreatAsAtomicUnit=on
  Dem_SetEventDisabled_Call4 : Subsystem  TreatAsAtomicUnit=on
  Dem_SetEventDisabled_Call5 : Subsystem  TreatAsAtomicUnit=on
  Dem_SetEventDisabled_Call6 : Subsystem  TreatAsAtomicUnit=on
  Dem_SetEventDisabled_Call7 : Subsystem  TreatAsAtomicUnit=on
  Dem_SetEventDisabled_Call8 : Subsystem  TreatAsAtomicUnit=on
  Demux : Demux  Outputs=9
  wires:
  set_flag/1 -> Demux/1  "set_flag"
  Demux/2 -> Dem_SetEventDisabled_Call1/Enable  "set_flag1"
  Demux/3 -> Dem_SetEventDisabled_Call2/Enable  "set_flag2"
  Demux/4 -> Dem_SetEventDisabled_Call3/Enable  "set_flag3"
  Demux/5 -> Dem_SetEventDisabled_Call4/Enable  "set_flag4"
  Demux/6 -> Dem_SetEventDisabled_Call5/Enable  "set_flag5"
  Demux/7 -> Dem_SetEventDisabled_Call6/Enable  "set_flag6"
  Demux/8 -> Dem_SetEventDisabled_Call7/Enable  "set_flag7"
  Demux/9 -> Dem_SetEventDisabled_Call8/Enable  "set_flag8"
  Demux/1 -> Dem_SetEventDisabled_Call0/Enable  "set_flag0"

== system AEMS_Standard_Library/SUB/AEMS_DEM_SET_EVENT_STS_1D ==
  diag_set_input_flag : Inport  PortDimensions=1
  AEMS_EDGE_RISING : AEMS_Standard_Library/EDGE/AEMS_EDGE_RISING  Tag=[LIB]  init=false
      settings: AttributesFormatString=|
      | %<MaskType>
      | Initial Value : %<init>
  Dem_SetEventStatus_Call : Subsystem  TreatAsAtomicUnit=on
  dgn_event_status_failed : Constant  OutDataTypeStr=uint8
  wires:
  dgn_event_status_failed/1 -> Dem_SetEventStatus_Call/1(dem_event_status_failed)  "dem_event_status_failed"
  diag_set_input_flag/1 -> AEMS_EDGE_RISING/1  "diag_set_input_flag"
  AEMS_EDGE_RISING/1 -> Dem_SetEventStatus_Call/Enable  "trigger_job_1st"

== system AEMS_Standard_Library/SUB/AEMS_DEM_SET_EVENT_STS_2D ==
  diag_set_input_flag : Inport
  AEMS_EDGE_RISING : AEMS_Standard_Library/EDGE/AEMS_EDGE_RISING  Tag=[LIB]  init=false
      settings: AttributesFormatString=|
      | %<MaskType>
      | Initial Value : %<init>
  AEMS_EDGE_RISING1 : AEMS_Standard_Library/EDGE/AEMS_EDGE_RISING  Tag=[LIB]  init=false
      settings: AttributesFormatString=|
      | %<MaskType>
      | Initial Value : %<init>
  Dem_SetEventStatus_Call1 : Subsystem  TreatAsAtomicUnit=on
  Dem_SetEventStatus_Call2 : Subsystem  TreatAsAtomicUnit=on
  Demux : Demux  Outputs=2
  dgn_event_status_failed1 : Constant  OutDataTypeStr=uint8
  dgn_event_status_failed2 : Constant  OutDataTypeStr=uint8
  wires:
  diag_set_input_flag/1 -> Demux/1  "diag_set_input_flag"
  dgn_event_status_failed1/1 -> Dem_SetEventStatus_Call1/1(dem_event_status_failed1)  "dem_event_status_failed1"
  Demux/1 -> AEMS_EDGE_RISING/1  "diag_set_input_flag1"
  dgn_event_status_failed2/1 -> Dem_SetEventStatus_Call2/1(dem_event_status_failed2)  "dem_event_status_failed2"
  Demux/2 -> AEMS_EDGE_RISING1/1  "diag_set_input_flag2"
  AEMS_EDGE_RISING/1 -> Dem_SetEventStatus_Call1/Enable  "trigger_job_1st1"
  AEMS_EDGE_RISING1/1 -> Dem_SetEventStatus_Call2/Enable  "trigger_job_1st2"

== system AEMS_Standard_Library/SUB/AEMS_DEM_SET_EVENT_STS_8D ==
  diag_set_input_flag : Inport
  AEMS_EDGE_RISING{,1..7} (8 alike) : AEMS_Standard_Library/EDGE/AEMS_EDGE_RISING  Tag=[LIB]  init=false
      settings: AttributesFormatString=|
      | %<MaskType>
      | Initial Value : %<init>
  Dem_SetEventStatus_Call1 : Subsystem  TreatAsAtomicUnit=on
  Dem_SetEventStatus_Call2 : Subsystem  TreatAsAtomicUnit=on
  Dem_SetEventStatus_Call3 : Subsystem  TreatAsAtomicUnit=on
  Dem_SetEventStatus_Call4 : Subsystem  TreatAsAtomicUnit=on
  Dem_SetEventStatus_Call5 : Subsystem  TreatAsAtomicUnit=on
  Dem_SetEventStatus_Call6 : Subsystem  TreatAsAtomicUnit=on
  Dem_SetEventStatus_Call7 : Subsystem  TreatAsAtomicUnit=on
  Dem_SetEventStatus_Call8 : Subsystem  TreatAsAtomicUnit=on
  Demux : Demux  Outputs=8
  dgn_event_status_failed{1..8} (8 alike) : Constant  OutDataTypeStr=uint8
  wires:
  dgn_event_status_failed1/1 -> Dem_SetEventStatus_Call1/1(dem_event_status_failed1)  "dem_event_status_failed1"
  diag_set_input_flag/1 -> Demux/1  "diag_set_input_flag"
  Demux/1 -> AEMS_EDGE_RISING/1  "diag_set_input_flag1"
  dgn_event_status_failed2/1 -> Dem_SetEventStatus_Call2/1(dem_event_status_failed2)  "dem_event_status_failed2"
  Demux/2 -> AEMS_EDGE_RISING1/1  "diag_set_input_flag2"
  dgn_event_status_failed3/1 -> Dem_SetEventStatus_Call3/1(dem_event_status_failed3)  "dem_event_status_failed3"
  Demux/3 -> AEMS_EDGE_RISING2/1  "diag_set_input_flag3"
  dgn_event_status_failed4/1 -> Dem_SetEventStatus_Call4/1(dem_event_status_failed4)  "dem_event_status_failed4"
  Demux/4 -> AEMS_EDGE_RISING3/1  "diag_set_input_flag4"
  dgn_event_status_failed5/1 -> Dem_SetEventStatus_Call5/1(dem_event_status_failed5)  "dem_event_status_failed5"
  Demux/5 -> AEMS_EDGE_RISING4/1  "diag_set_input_flag5"
  dgn_event_status_failed6/1 -> Dem_SetEventStatus_Call6/1(dem_event_status_failed6)  "dem_event_status_failed6"
  Demux/6 -> AEMS_EDGE_RISING5/1  "diag_set_input_flag6"
  dgn_event_status_failed7/1 -> Dem_SetEventStatus_Call7/1(dem_event_status_failed7)  "dem_event_status_failed7"
  Demux/7 -> AEMS_EDGE_RISING6/1  "diag_set_input_flag7"
  Demux/8 -> AEMS_EDGE_RISING7/1  "diag_set_input_flag8"
  dgn_event_status_failed8/1 -> Dem_SetEventStatus_Call8/1(dem_event_status_failed8)  "dem_event_status_failed8"
  AEMS_EDGE_RISING/1 -> Dem_SetEventStatus_Call1/Enable  "trigger_job_1st1"
  AEMS_EDGE_RISING1/1 -> Dem_SetEventStatus_Call2/Enable  "trigger_job_1st2"
  AEMS_EDGE_RISING2/1 -> Dem_SetEventStatus_Call3/Enable  "trigger_job_1st3"
  AEMS_EDGE_RISING3/1 -> Dem_SetEventStatus_Call4/Enable  "trigger_job_1st4"
  AEMS_EDGE_RISING4/1 -> Dem_SetEventStatus_Call5/Enable  "trigger_job_1st5"
  AEMS_EDGE_RISING5/1 -> Dem_SetEventStatus_Call6/Enable  "trigger_job_1st6"
  AEMS_EDGE_RISING6/1 -> Dem_SetEventStatus_Call7/Enable  "trigger_job_1st7"
  AEMS_EDGE_RISING7/1 -> Dem_SetEventStatus_Call8/Enable  "trigger_job_1st8"

== system AEMS_Standard_Library/SUB/AEMS_DEM_SET_EVENT_STS_9D ==
  diag_set_input_flag : Inport  OutDataTypeStr=boolean  PortDimensions=9
      settings: AttributesFormatString=<tsample=%<SampleTime>>
  AEMS_EDGE_RISING{,1..8} (9 alike) : AEMS_Standard_Library/EDGE/AEMS_EDGE_RISING  Tag=[LIB]  init=false
      settings: AttributesFormatString=|
      | %<MaskType>
      | Initial Value : %<init>
  Dem_SetEventStatus_Call0 : Subsystem  TreatAsAtomicUnit=on
  Dem_SetEventStatus_Call1 : Subsystem  TreatAsAtomicUnit=on
  Dem_SetEventStatus_Call2 : Subsystem  TreatAsAtomicUnit=on
  Dem_SetEventStatus_Call3 : Subsystem  TreatAsAtomicUnit=on
  Dem_SetEventStatus_Call4 : Subsystem  TreatAsAtomicUnit=on
  Dem_SetEventStatus_Call5 : Subsystem  TreatAsAtomicUnit=on
  Dem_SetEventStatus_Call6 : Subsystem  TreatAsAtomicUnit=on
  Dem_SetEventStatus_Call7 : Subsystem  TreatAsAtomicUnit=on
  Dem_SetEventStatus_Call8 : Subsystem  TreatAsAtomicUnit=on
  Demux : Demux  Outputs=9
  dgn_event_status_failed{0..8} (9 alike) : Constant  OutDataTypeStr=uint8
  wires:
  AEMS_EDGE_RISING8/1 -> Dem_SetEventStatus_Call8/Enable  "trigger_job_1st8"
  AEMS_EDGE_RISING7/1 -> Dem_SetEventStatus_Call7/Enable  "trigger_job_1st7"
  AEMS_EDGE_RISING6/1 -> Dem_SetEventStatus_Call6/Enable  "trigger_job_1st6"
  AEMS_EDGE_RISING5/1 -> Dem_SetEventStatus_Call5/Enable  "trigger_job_1st5"
  AEMS_EDGE_RISING4/1 -> Dem_SetEventStatus_Call4/Enable  "trigger_job_1st4"
  AEMS_EDGE_RISING3/1 -> Dem_SetEventStatus_Call3/Enable  "trigger_job_1st3"
  AEMS_EDGE_RISING2/1 -> Dem_SetEventStatus_Call2/Enable  "trigger_job_1st2"
  AEMS_EDGE_RISING1/1 -> Dem_SetEventStatus_Call1/Enable  "trigger_job_1st1"
  dgn_event_status_failed8/1 -> Dem_SetEventStatus_Call8/1(dem_event_status_failed8)  "dem_event_status_failed8"
  dgn_event_status_failed7/1 -> Dem_SetEventStatus_Call7/1(dem_event_status_failed7)  "dem_event_status_failed7"
  dgn_event_status_failed6/1 -> Dem_SetEventStatus_Call6/1(dem_event_status_failed6)  "dem_event_status_failed6"
  dgn_event_status_failed5/1 -> Dem_SetEventStatus_Call5/1(dem_event_status_failed5)  "dem_event_status_failed5"
  dgn_event_status_failed4/1 -> Dem_SetEventStatus_Call4/1(dem_event_status_failed4)  "dem_event_status_failed4"
  dgn_event_status_failed3/1 -> Dem_SetEventStatus_Call3/1(dem_event_status_failed3)  "dem_event_status_failed3"
  dgn_event_status_failed2/1 -> Dem_SetEventStatus_Call2/1(dem_event_status_failed2)  "dem_event_status_failed2"
  diag_set_input_flag/1 -> Demux/1  "diag_set_input_flag"
  dgn_event_status_failed1/1 -> Dem_SetEventStatus_Call1/1(dem_event_status_failed1)  "dem_event_status_failed1"
  AEMS_EDGE_RISING/1 -> Dem_SetEventStatus_Call0/Enable  "trigger_job_1st0"
  Demux/1 -> AEMS_EDGE_RISING/1  "diag_set_input_flag0"
  dgn_event_status_failed0/1 -> Dem_SetEventStatus_Call0/1(dem_event_status_failed0)  "dem_event_status_failed0"
  Demux/2 -> AEMS_EDGE_RISING1/1  "diag_set_input_flag1"
  Demux/3 -> AEMS_EDGE_RISING2/1  "diag_set_input_flag2"
  Demux/4 -> AEMS_EDGE_RISING3/1  "diag_set_input_flag3"
  Demux/5 -> AEMS_EDGE_RISING4/1  "diag_set_input_flag4"
  Demux/6 -> AEMS_EDGE_RISING5/1  "diag_set_input_flag5"
  Demux/7 -> AEMS_EDGE_RISING6/1  "diag_set_input_flag6"
  Demux/8 -> AEMS_EDGE_RISING7/1  "diag_set_input_flag7"
  Demux/9 -> AEMS_EDGE_RISING8/1  "diag_set_input_flag8"

== system AEMS_Standard_Library/SUB/AEMS_DEM_SET_STORAGE_COND_1D ==
  conditionfulfilled : Inport
  AEMS_DEM_SETSTORAGECONDITION : AEMS_Standard_Library/SUB/AEMS_DEM_SETSTORAGECONDITION  Tag=[LIB]
      settings: AttributesFormatString=%<MaskType>
  StorageCondId_block : Constant  Value=Dem_StorageConditionId_XXX  OutDataTypeStr=uint8
  wires:
  StorageCondId_block/1 -> AEMS_DEM_SETSTORAGECONDITION/1  "storageconditionid"
  conditionfulfilled/1 -> AEMS_DEM_SETSTORAGECONDITION/2  "conditionfulfilled"

== system AEMS_Standard_Library/SUB/AEMS_DEM_SET_STORAGE_COND_2D ==
  conditionfulfilled : Inport
  AEMS_DEM_SETSTORAGECONDITION1 : AEMS_Standard_Library/SUB/AEMS_DEM_SETSTORAGECONDITION  Tag=[LIB]
      settings: AttributesFormatString=%<MaskType>
  AEMS_DEM_SETSTORAGECONDITION2 : AEMS_Standard_Library/SUB/AEMS_DEM_SETSTORAGECONDITION  Tag=[LIB]
      settings: AttributesFormatString=%<MaskType>
  Demux1 : Demux  Outputs=2
  StorageConditionId_block1 : Constant  Value=Dem_StorageConditionId_XXX  OutDataTypeStr=uint8
  StorageConditionId_block2 : Constant  Value=Dem_StorageConditionId2_XXX  OutDataTypeStr=uint8
  wires:
  conditionfulfilled/1 -> Demux1/1  "conditionfulfilled"
  Demux1/1 -> AEMS_DEM_SETSTORAGECONDITION1/2  "conditionfulfilled1"
  StorageConditionId_block1/1 -> AEMS_DEM_SETSTORAGECONDITION1/1  "storageconditionid1"
  StorageConditionId_block2/1 -> AEMS_DEM_SETSTORAGECONDITION2/1  "storageconditionid2"
  Demux1/2 -> AEMS_DEM_SETSTORAGECONDITION2/2  "conditionfulfilled2"
